simulink model "respuestademotor"  (Simulink 7.5)
settings: Solver=ode45  StartTime=0.0  StopTime=10.0  RelTol=1e-3
settings Model: Creator=My Laptop  LastModifiedBy=Mariano

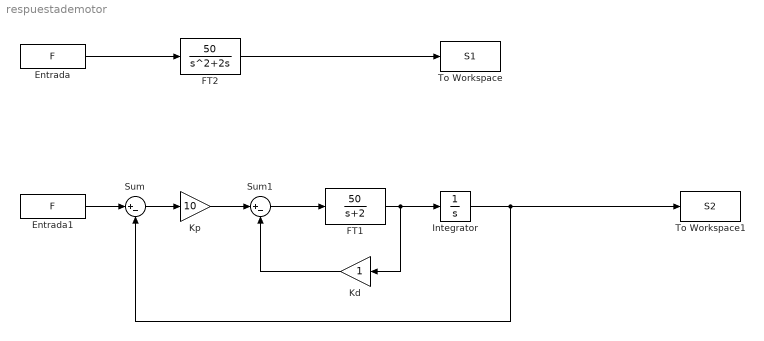
== system respuestademotor ==
  Entrada : FromWorkspace  VariableName=F  SampleTime=0.01  OutputAfterFinalValue=Holding final value
  Entrada1 : FromWorkspace  VariableName=F  SampleTime=0.01  OutputAfterFinalValue=Holding final value
  FT1 : TransferFcn  Numerator=[50]  Denominator=[1 2]
  FT2 : TransferFcn  Numerator=[50]  Denominator=[1 2 0]
  Integrator : Integrator
  Kd : Gain  ParameterDataType=fixdt(1, 16)  ParameterScaling=2^0  OutDataType=fixdt(1, 16)  OutScaling=2^0
  Kp : Gain  Gain=10  ParameterDataType=fixdt(1, 16)  ParameterScaling=2^0  OutDataType=fixdt(1, 16)  OutScaling=2^0
  Sum : Sum  Inputs=|+-  OutDataType=fixdt(1, 16)  OutScaling=2^0
  Sum1 : Sum  Inputs=|+-  OutDataType=fixdt(1, 16)  OutScaling=2^0
  To Workspace : ToWorkspace  VariableName=S1  SampleTime=-1  SaveFormat=Array
  To Workspace1 : ToWorkspace  VariableName=S2  SampleTime=-1  SaveFormat=Array
  wires:
  Entrada/1 -> FT2/1
  FT2/1 -> To Workspace/1
  FT1/1 -> Integrator/1, Kd/1
  Sum1/1 -> FT1/1
  Kp/1 -> Sum1/1
  Sum/1 -> Kp/1
  Integrator/1 -> Sum/2, To Workspace1/1
  Entrada1/1 -> Sum/1
  Kd/1 -> Sum1/2
